simulink model "simulacion_ejercicio1_vertical"  (R2024a)
settings: Solver=FixedStepAuto  StartTime=0.0  StopTime=9  FixedStep=0.001  RelTol=1e-3
values from neighbouring files (symbols this model uses):
  a_adelanto = y + real_Pd1    [ejercicio1_vertical.m]
  a_retraso = 0.01    [ejercicio1_vertical.m]
  b_adelanto = abs(real(Pd1))    [ejercicio1_vertical.m]
  b_retraso = (Kv_deseado*a_retraso*a_adelanto*50)/(K_rlocfind*real_Pd1*25)    [ejercicio1_vertical.m]
  final_escalon = 1    [ejercicio1_vertical.m]
  K_retraso = 1    [ejercicio1_vertical.m]
  Mp = 4.33/100    (= 0.0433)    [ejercicio1_vertical.m]
undefined symbols (not defined in the file or in its folder): K_rlocfind
libraries: simulink x1
settings Model: Creator=david  LastModifiedBy=david

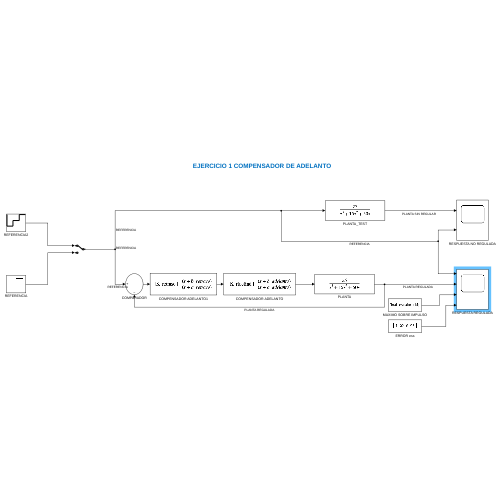
[thumbnail: Simulink's stored preview of the top-level diagram]
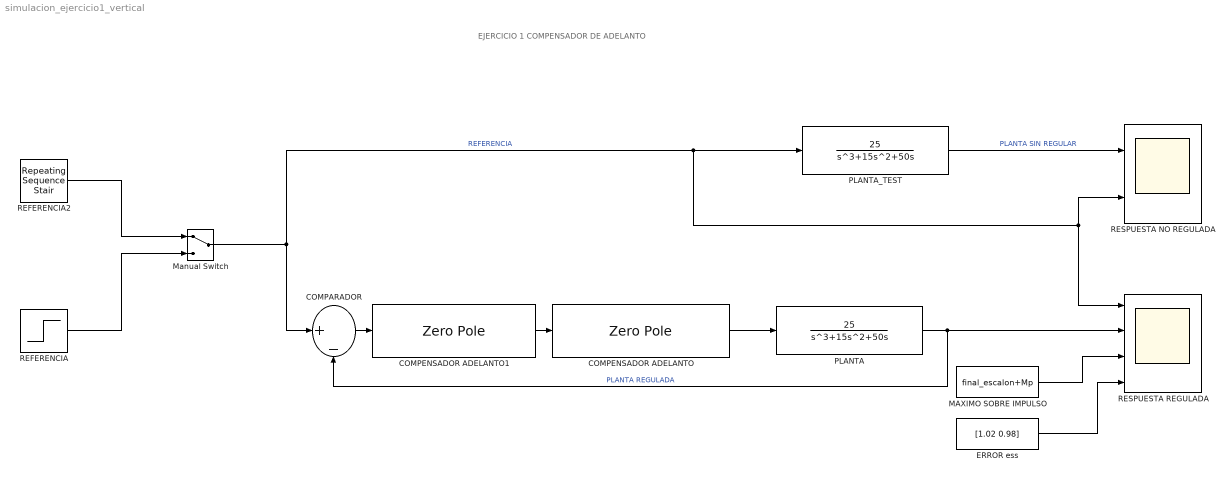
== system simulacion_ejercicio1_vertical ==
  note: EJERCICIO 1 COMPENSADOR DE ADELANTO
  COMPARADOR : Sum  Inputs=|+-
  COMPENSADOR ADELANTO : ZeroPole  Zeros=[-b_adelanto]  Poles=[-a_adelanto]  Gain=[K_rlocfind]
  COMPENSADOR ADELANTO1 : ZeroPole  Zeros=[-b_retraso]  Poles=[-a_retraso]  Gain=[K_retraso]
  ERROR ess : Constant  Value=[1.02 0.98]
  MAXIMO SOBRE IMPULSO : Constant  Value=final_escalon+Mp
  Manual Switch : ManualSwitch
  PLANTA : TransferFcn  Numerator=[25]  Denominator=[1 15 50 0]
  PLANTA_TEST : TransferFcn  Numerator=[25]  Denominator=[1 15 50 0]
  REFERENCIA : Step  After=final_escalon  SampleTime=0
  REFERENCIA2 : simulink/Sources/Repeating Sequence Stair  OutValues=[1 2 3]  tsamp=3  OutMin=[]  OutMax=[]  OutDataTypeStr=double  OutputDataTypeScalingMode=double  OutDataType=fixdt(0,8)  ConRadixGroup=Best Precision: Vector-wise  OutScaling=2^-12
  RESPUESTA NO REGULADA : Scope  NumInputPorts=2
  RESPUESTA REGULADA : Scope  NumInputPorts=4
  wires:
  Manual Switch/1 -> PLANTA_TEST/1, RESPUESTA NO REGULADA/2, RESPUESTA REGULADA/1, COMPARADOR/1  "REFERENCIA"
  COMPENSADOR ADELANTO/1 -> PLANTA/1
  PLANTA/1 -> RESPUESTA REGULADA/2, COMPARADOR/2  "PLANTA REGULADA"
  PLANTA_TEST/1 -> RESPUESTA NO REGULADA/1  "PLANTA SIN REGULAR"
  MAXIMO SOBRE IMPULSO/1 -> RESPUESTA REGULADA/3
  ERROR ess/1 -> RESPUESTA REGULADA/4
  REFERENCIA2/1 -> Manual Switch/1
  REFERENCIA/1 -> Manual Switch/2
  COMPARADOR/1 -> COMPENSADOR ADELANTO1/1
  COMPENSADOR ADELANTO1/1 -> COMPENSADOR ADELANTO/1
